simulink model "OFDME"  (R2020b)
settings: Solver=VariableStepAuto  StartTime=0.0  StopTime=inf  RelTol=1e-3
PreLoadFcn:
  | N = 64;
  | TsOFDM = 0.1e-6;
InitFcn:
  | N = 64;
  | TsOFDM = 0.1e-6;
undefined symbols (not defined in the file or in its folder): doppler
libraries: dspxfrm3 x2, dspindex x2, commdigbbndpm3 x2, commrandsrc3 x1, commsink2 x1, commchan3 x1
settings Model: SimulationMode=accelerator  Creator=t_issarni  LastModifiedBy=ncavalier

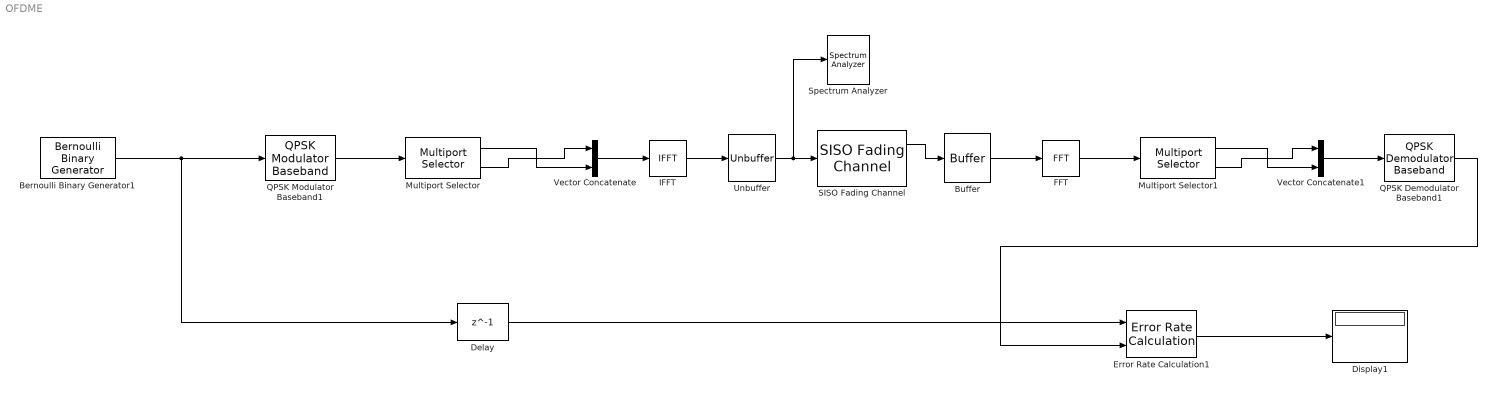
== system OFDME ==
  Bernoulli Binary Generator1 : commrandsrc3/Bernoulli Binary Generator  ProbabilityOfZero=0.5  SeedSource=Parameter  Seed=randi(100)  SampleTime=TsOFDM/(2*N)  SamplesPerFrame=2*N  OutputDataType=double  SimulateUsing=Code generation
  Buffer : Buffer  OutputFrames=off
  Delay : Delay  DelayLength=1  InitialCondition=0  UseCircularBuffer=on
  Display1 : Display
  Error Rate Calculation1 : commsink2/Error Rate Calculation  N=0  st_delay=0  cp_mode=Entire frame  subframe=[]  PMode=Port  WsName=ErrorVec  RsMode2=off  stop=off  numErr=100  maxBits=1e6
      settings: SourceProductName=Communications Toolbox
  FFT : dspxfrm3/FFT  FFTImplementation=Auto  CompMethod=Table lookup  TableOpt=NEW  TableOptActive=Speed  BitRevOrder=off  Normalize=off  InheritFFTLength=on  FFTLength=64  WrapInput=on  roundingMode=Floor  overflowMode=off  firstCoeffDataTypeStr=Inherit: Same word length as input  firstCoeffLastDataTypeStr=Inherit: Same word length as input  outputMin=[]  outputMax=[]
  IFFT : dspxfrm3/IFFT  FFTImplementation=Auto  CompMethod=Table lookup  TableOpt=NEW  TableOptActive=Speed  BitRevOrder=off  cs_in=off  Normalize=on  InheritFFTLength=on  FFTLength=64  WrapInput=on  mode=Complex  outSamplingMode=Sample based  roundingMode=Floor  overflowMode=off  firstCoeffDataTypeStr=Inherit: Same word length as input  firstCoeffLastDataTypeStr=Inherit: Same word length as input  outputMin=[]  outputMax=[]
  Multiport Selector : dspindex/Multiport Selector  rowsOrCols=Rows  idxCellArray={1 : N/2, (N/2)+1 : N }  idxErrMode=Clip Index
  Multiport Selector1 : dspindex/Multiport Selector  rowsOrCols=Rows  idxCellArray={1 : N/2, (N/2)+1 : N }  idxErrMode=Clip Index
  QPSK Demodulator Baseband1 : commdigbbndpm3/QPSK Demodulator Baseband  OutType=Bit  DecType=Hard decision  VarSource=Dialog  Variance=1  Dec=Gray  Ph=pi/4  outDtype1=Inherit via internal rule  outDtype2=Inherit via internal rule  derotateFactorWordLen=16  derotateFactorDataTypeStr=Inherit: Same word length as input  derotateFactorLastDataTypeStr=Inherit: Same word length as input
      settings: SourceProductName=Communications Toolbox
  QPSK Modulator Baseband1 : commdigbbndpm3/QPSK Modulator Baseband  InType=Bit  Enc=Gray  Ph=pi/4  outDtype=double  outWordLen=16  outUDDataType=sfix(16)  outFracLenMode=Best precision  outFracLen=15  outDataTypeStr=double  outLastDataTypeStr=double
      settings: SourceProductName=Communications Toolbox
  SISO Fading Channel : commchan3/SISO Fading Channel  InheritSampleRate=on  SampleRate=1  PathDelays=[0 TsOFDM/N]  AveragePathGains=[0 -3]  NormalizePathGains=on  FadingDistribution=Rayleigh  KFactor=3  DirectPathDopplerShift=0  DirectPathInitialPhase=0  MaximumDopplerShift=0  DopplerSpectrum=doppler('Jakes')  RandomStream=mt19937ar with seed  Seed=randi(100)  PathGainsOutputPort=on  ChannelFilterDelayOutputPort=off  SimulateUsing=Code generation  Visualization=Off  PathsForDopplerDisplay=1  SamplesToDisplay=25%
  Spectrum Analyzer : SpectrumAnalyzer
  Unbuffer : Unbuffer
  Vector Concatenate : Concatenate
  Vector Concatenate1 : Concatenate
  wires:
  Error Rate Calculation1/1 -> Display1/1
  QPSK Demodulator Baseband1/1 -> Error Rate Calculation1/2
  QPSK Modulator Baseband1/1 -> Multiport Selector/1
  Multiport Selector/2 -> Vector Concatenate/1
  Multiport Selector/1 -> Vector Concatenate/2
  Vector Concatenate/1 -> IFFT/1
  Vector Concatenate1/1 -> QPSK Demodulator Baseband1/1
  Multiport Selector1/2 -> Vector Concatenate1/1
  Multiport Selector1/1 -> Vector Concatenate1/2
  FFT/1 -> Multiport Selector1/1
  Buffer/1 -> FFT/1
  IFFT/1 -> Unbuffer/1
  Bernoulli Binary Generator1/1 -> Delay/1, QPSK Modulator Baseband1/1
  Delay/1 -> Error Rate Calculation1/1
  Unbuffer/1 -> Spectrum Analyzer/1, SISO Fading Channel/1
  SISO Fading Channel/1 -> Buffer/1
